simulink model "untitled"  (R2020a)
settings: Solver=VariableStepAuto  StartTime=0.0  StopTime=100  RelTol=1e-3
settings Model: Creator=dinhm  LastModifiedBy=dinhm

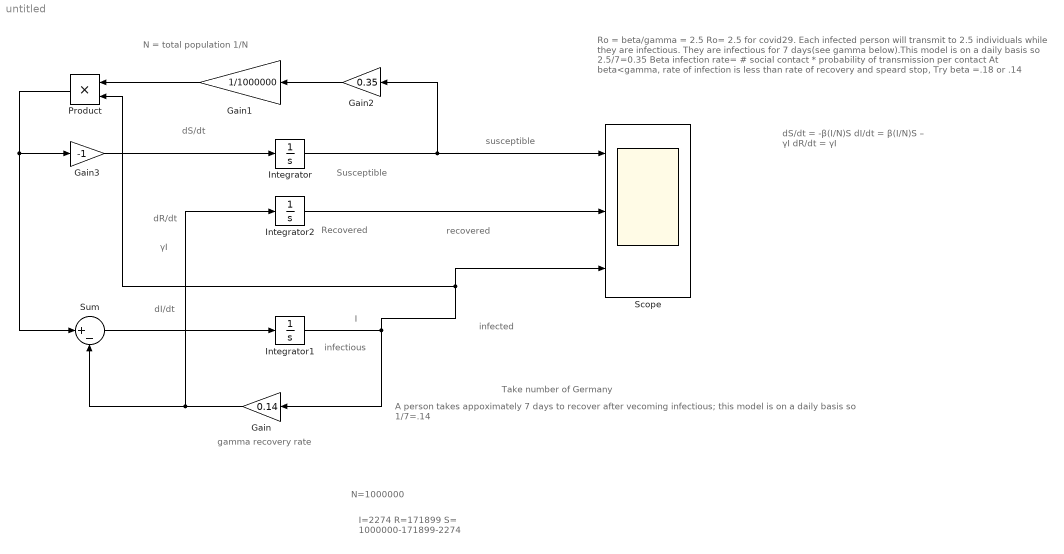
== system untitled ==
  note: I=2274
      | R=171899
      | S= 1000000-171899-2274
  note: N=1000000
  note: Take number of Germany
  note: A person takes appoximately 7 days to recover after vecoming infectious; this model is on a daily basis so 1/7=.14
  note: I
  note: γI
  note: susceptible
  note: Susceptible
  note: recovered
  note: Recovered
  note: infectious
  note: gamma recovery rate
  note: infected
  note: dI/dt
  note: dR/dt
  note: dS/dt
  note: dS/dt = -β(I/N)S
      | dI/dt = β(I/N)S – γI
      | dR/dt = γI
  note: Ro = beta/gamma = 2.5
      | Ro= 2.5 for covid29. Each infected person will transmit to 2.5 individuals while they are infectious.
      | They are infectious for 7 days(see gamma below).This model is on a daily basis so 2.5/7=0.35
      | Beta infection rate= # social contact * probability of transmission per contact
      |
      | At beta<gamma, rate of infection is less than rate of recovery and speard stop, Try beta =.18 or .14
  note: N = total population 1/N
  Gain : Gain  Gain=0.14
  Gain1 : Gain  Gain=1/1000000
  Gain2 : Gain  Gain=0.35
  Gain3 : Gain  Gain=-1
  Integrator : Integrator  InitialCondition=1000000-171899-2274
  Integrator1 : Integrator  InitialCondition=2274
  Integrator2 : Integrator  InitialCondition=171899
  Product : Product
  Scope : Scope  NumInputPorts=3
  Sum : Sum  Inputs=|+-
  wires:
  Integrator2/1 -> Scope/2
  Integrator1/1 -> Gain/1, Scope/3, Product/2
  Gain1/1 -> Product/1
  Gain2/1 -> Gain1/1
  Integrator/1 -> Gain2/1, Scope/1
  Gain/1 -> Integrator2/1, Sum/2
  Sum/1 -> Integrator1/1
  Gain3/1 -> Integrator/1
  Product/1 -> Sum/1, Gain3/1
